simulink model "vesitankki"  (R2017b)
settings: Solver=VariableStepAuto  StartTime=0.0  StopTime=100  MaxStep=0.1  RelTol=1e-3
values from neighbouring files (symbols this model uses):
  A = 5    [kt.m]    (also in tehtava_b.m)
  D = 0    [kt.m]    (also in tehtava_b.m = 8)
  f = 0.01    [kt.m]
  f_in_orig = 20    [kt.m]    (also in tehtava_b.m)
  h0 = 100    [kt.m]    (also in tehtava_b.m)
  h_ref = 100    [kt.m]    (also in tehtava_b.m)
  I = 0    [kt.m]    (also in tehtava_b.m = 1)
  k_v = 2.0    (= 2)    [kt.m]    (also in tehtava_b.m)
  P = 0    [kt.m]    (also in tehtava_b.m = 15)
libraries: simulink x1
settings Model: Creator=Timo Järvinen  LastModifiedBy=Timo Järvinen

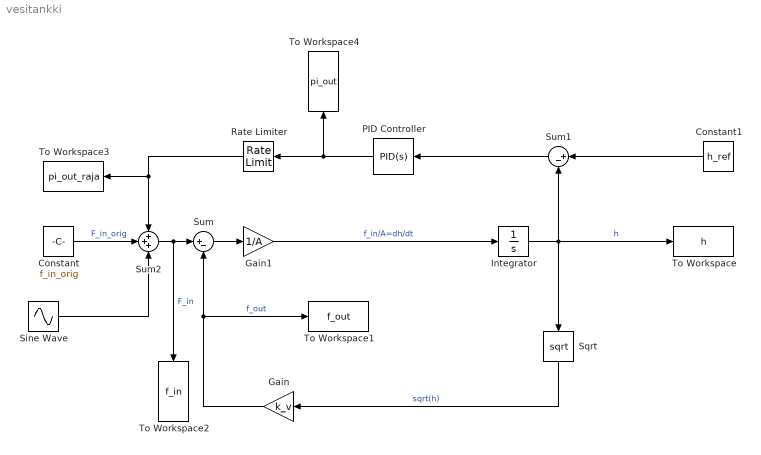
== system vesitankki ==
  Constant : Constant  Value=f_in_orig
  Constant1 : Constant  Value=h_ref
  Gain : Gain  Gain=k_v
  Gain1 : Gain  Gain=1/A
  Integrator : Integrator  InitialCondition=h0
  PID Controller : simulink/Continuous/PID Controller  Controller=PID  TimeDomain=Continuous-time  SampleTime=-1  IntegratorMethod=Forward Euler  FilterMethod=Forward Euler  Form=Parallel  UseFilter=on  ControllerParametersSource=internal  P=P  I=I  D=D  N=100  InitialConditionSource=internal  InitialConditionForIntegrator=0  InitialConditionForFilter=0  ExternalReset=none  LimitOutput=off  UpperSaturationLimit=inf  LowerSaturationLimit=-inf  LinearizeAsGain=on  AntiWindupMode=none  Kb=1  TrackingMode=off  Kt=1  PParamMin=[]  PParamMax=[]  IParamMin=[]  IParamMax=[]  DParamMin=[]  DParamMax=[]  NParamMin=[]  NParamMax=[]  KbParamMin=[]  KbParamMax=[]  KtParamMin=[]  KtParamMax=[]  POutMin=[]  POutMax=[]  IOutMin=[]  IOutMax=[]  DOutMin=[]  DOutMax=[]  NOutMin=[]  NOutMax=[]  KbOutMin=[]  KbOutMax=[]  KtOutMin=[]  KtOutMax=[]  IntegratorOutMin=[]  IntegratorOutMax=[]  FilterOutMin=[]  FilterOutMax=[]  SumOutMin=[]  SumOutMax=[]  SumI1OutMin=[]  SumI1OutMax=[]  SumI2OutMin=[]  SumI2OutMax=[]  SumI3OutMin=[]  SumI3OutMax=[]  SumDOutMin=[]  SumDOutMax=[]  SaturationOutMin=[]  SaturationOutMax=[]  IntegratorContinuousStateAttributes=''  IntegratorStateMustResolveToSignalObject=off  IntegratorRTWStateStorageClass=Auto  FilterContinuousStateAttributes=''  FilterStateMustResolveToSignalObject=off  FilterRTWStateStorageClass=Auto  DifferentiatorICPrevScaledInput=0  DifferentiatorOutMin=[]  DifferentiatorOutMax=[]  InitialConditionSetting=State (most efficient)  FilterDiffOutCoefMin=[]  FilterDiffOutCoefMax=[]  SumDenOutMin=[]  SumDenOutMax=[]  SumNumOutMin=[]  SumNumOutMax=[]  ReciprocalOutMin=[]  ReciprocalOutMax=[]  DivideOutMin=[]  DivideOutMax=[]  TunerSelectOption=Transfer Function Based (PID Tuner App)
  Rate Limiter : RateLimiter  RisingSlewLimit=5  SampleTimeMode=inherited
  Sine Wave : Sin  Frequency=f  SampleTime=0
  Sqrt : Sqrt  SaturateOnIntegerOverflow=on
  Sum : Sum  Inputs=|+-
  Sum1 : Sum  Inputs=|+-
  Sum2 : Sum  Inputs=+++
  To Workspace : ToWorkspace  VariableName=h  SampleTime=-1
  To Workspace1 : ToWorkspace  VariableName=f_out  SampleTime=-1
  To Workspace2 : ToWorkspace  VariableName=f_in  SampleTime=-1
  To Workspace3 : ToWorkspace  VariableName=pi_out_raja  SampleTime=-1
  To Workspace4 : ToWorkspace  VariableName=pi_out  SampleTime=-1
  wires:
  Integrator/1 -> Sum1/2, Sqrt/1, To Workspace/1  "h"
  Gain1/1 -> Integrator/1  "f_in/A=dh/dt"
  Sum/1 -> Gain1/1
  Sqrt/1 -> Gain/1  "sqrt(h)"
  Gain/1 -> To Workspace1/1, Sum/2  "f_out"
  Constant/1 -> Sum2/2  "F_in_orig"
  Sine Wave/1 -> Sum2/3
  Sum2/1 -> To Workspace2/1, Sum/1  "F_in"
  Sum1/1 -> PID Controller/1
  Constant1/1 -> Sum1/1
  PID Controller/1 -> To Workspace4/1, Rate Limiter/1
  Rate Limiter/1 -> To Workspace3/1, Sum2/1
